simulink library "motor_interface_lib"  (R2022b)
settings: Solver=VariableStepAuto  StartTime=0.0  StopTime=10.0  RelTol=1e-3
settings Model: Creator=dr_pa  LastModifiedBy=dr_pa

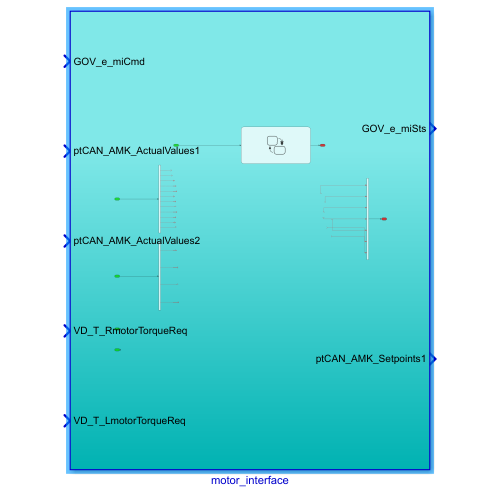
[thumbnail: Simulink's stored preview of the top-level diagram]
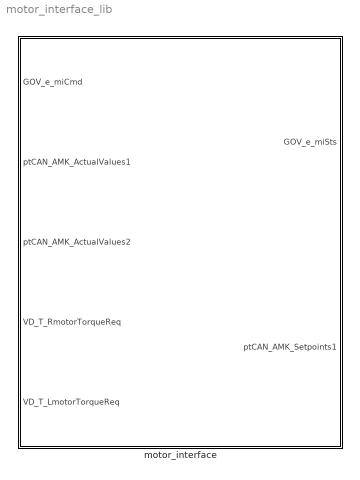
== system motor_interface_lib ==
  motor_interface : Subsystem

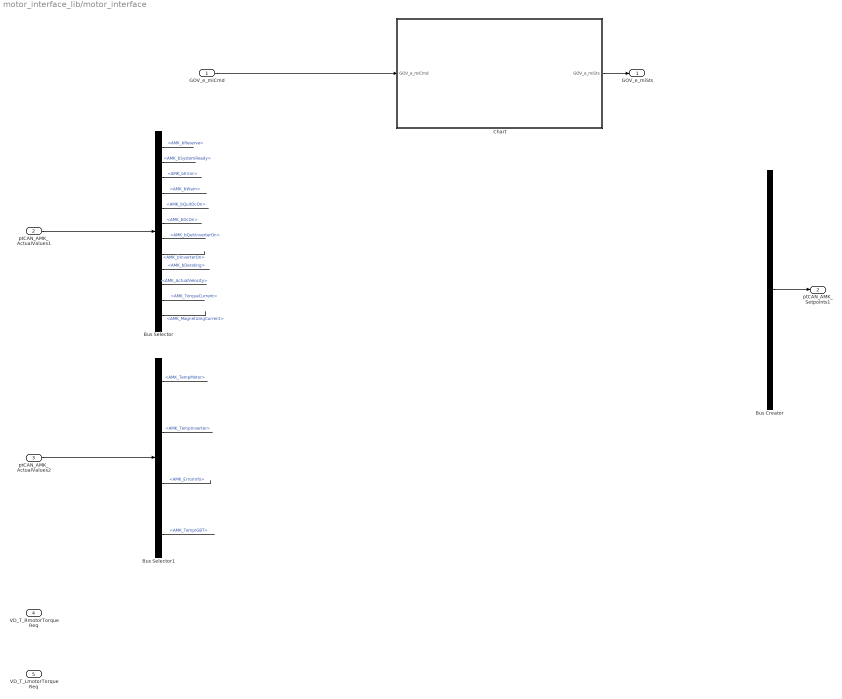
== system motor_interface_lib/motor_interface ==
  GOV_e_miCmd : Inport
  ptCAN_AMK_ActualValues1 : Inport  Port=2
  ptCAN_AMK_ActualValues2 : Inport  Port=3
  VD_T_RmotorTorqueReq : Inport  Port=4
  VD_T_LmotorTorqueReq : Inport  Port=5
  Bus Creator : BusCreator  Inputs=7
  Bus Selector : BusSelector  OutputSignals=AMK_bReserve,AMK_bSystemReady,AMK_bError,AMK_bWarn,AMK_bQuitDcOn,AMK_bDcOn,AMK_bQuitInverterOn,AMK_bInverterOn,AMK_bDerating,AMK_ActualVelocity,AMK_TorqueCurrent,AMK_MagnetizingCurrent
  Bus Selector1 : BusSelector  OutputSignals=AMK_TempMotor,AMK_TempInverter,AMK_ErrorInfo,AMK_TempIGBT
  Chart : Stateflow chart  TreatAsAtomicUnit=on
  GOV_e_miSts : Outport
  ptCAN_AMK_Setpoints1 : Outport  Port=2
  wires:
  GOV_e_miCmd/1 -> Chart/1(GOV_e_miCmd)
  Chart/1(GOV_e_miSts) -> GOV_e_miSts/1
  ptCAN_AMK_ActualValues1/1 -> Bus Selector/1
  Bus Selector/2 -> ?  "<AMK_bSystemReady>"
  Bus Selector/3 -> ?  "<AMK_bError>"
  Bus Selector/4 -> ?  "<AMK_bWarn>"
  Bus Selector/5 -> ?  "<AMK_bQuitDcOn>"
  Bus Selector/6 -> ?  "<AMK_bDcOn>"
  Bus Selector/7 -> ?  "<AMK_bQuitInverterOn>"
  Bus Selector/8 -> ?  "<AMK_bInverterOn>"
  Bus Selector/9 -> ?  "<AMK_bDerating>"
  Bus Selector/10 -> ?  "<AMK_ActualVelocity>"
  Bus Selector/11 -> ?  "<AMK_TorqueCurrent>"
  Bus Selector/12 -> ?  "<AMK_MagnetizingCurrent>"
  Bus Selector/1 -> ?  "<AMK_bReserve>"
  ptCAN_AMK_ActualValues2/1 -> Bus Selector1/1
  Bus Selector1/1 -> ?  "<AMK_TempMotor>"
  Bus Selector1/2 -> ?  "<AMK_TempInverter>"
  Bus Selector1/3 -> ?  "<AMK_ErrorInfo>"
  Bus Selector1/4 -> ?  "<AMK_TempIGBT>"
  Bus Creator/1 -> ptCAN_AMK_Setpoints1/1
  ? -> Bus Creator/1  "AMK_bInverterOn"
  ? -> Bus Creator/7  "AMK_TorqueLimitNegativ"
  ? -> Bus Creator/3  "AMK_bEnable"
  ? -> Bus Creator/5  "AMK_TargetVelocity"
  ? -> Bus Creator/2  "AMK_bDcOn"
  ? -> Bus Creator/4  "AMK_bErrorReset"
  ? -> Bus Creator/6  "AMK_TorqueLimitPositiv"

== stateflow chart motor_interface_lib/motor_interface/Chart ==
  data: GOV_e_miCmd input; GOV_e_miSts output
